simulink model "OfficeChairIntegratorsElekT4MarcelM"  (R2023a)
settings: Solver=VariableStepAuto  StartTime=0.0  StopTime=10.0  RelTol=1e-3
values from neighbouring files (symbols this model uses):
  C = 100*1e-6    (= 0.0001)    [SimOfficeChairIntegratorsT4MarcelM.m]
  g = 9.82    [SimOfficeChairIntegratorsT4MarcelM.m]
  L = 1.5*1e-6    (= 1.5e-06)    [SimOfficeChairIntegratorsT4MarcelM.m]
  M = 75    [SimOfficeChairIntegratorsT4MarcelM.m]
  Rx = 5e-2    (= 0.05)    [SimOfficeChairIntegratorsT4MarcelM.m]
settings Model: Creator=marcelmartens  LastModifiedBy=ullos

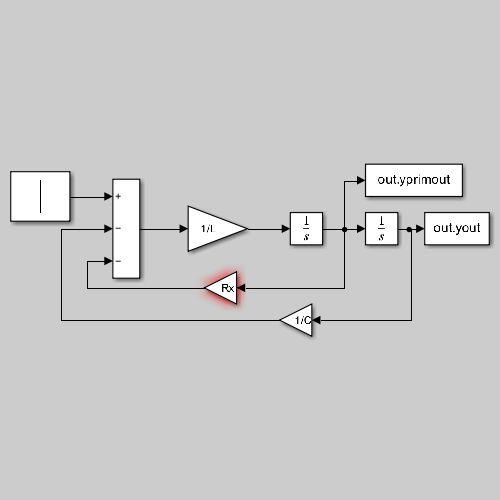
[thumbnail: Simulink's stored preview of the top-level diagram]
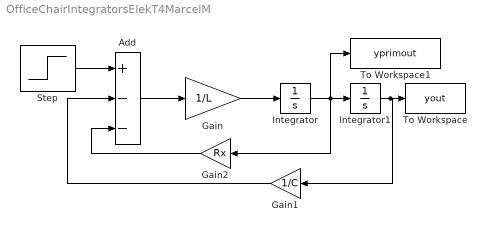
== system OfficeChairIntegratorsElekT4MarcelM ==
  Add : Sum  Inputs=+--
  Gain : Gain  Gain=1/L
  Gain1 : Gain  Gain=1/C
  Gain2 : Gain  Gain=Rx
  Integrator : Integrator
  Integrator1 : Integrator
  Step : Step  Time=0  After=M*g  SampleTime=0
  To Workspace : ToWorkspace  VariableName=yout  SaveFormat=Timeseries  SampleTime=-1
  To Workspace1 : ToWorkspace  VariableName=yprimout  SaveFormat=Timeseries  SampleTime=-1
  wires:
  Integrator1/1 -> To Workspace/1, Gain1/1
  Integrator/1 -> To Workspace1/1, Gain2/1, Integrator1/1
  Step/1 -> Add/1
  Gain1/1 -> Add/2
  Gain/1 -> Integrator/1
  Gain2/1 -> Add/3
  Add/1 -> Gain/1
